simulink model "LKA"  (Simulink 7.9)
settings: Solver=ode23  StartTime=0.0  StopTime=tend  FixedStep=0.01  RelTol=1e-3
undefined symbols (not defined in the file or in its folder): pin
libraries: library x6, simulink x3
settings Model: Creator=Georg  LastModifiedBy=georgnestlinger
settings OptimizationCC: InlineParams=on
settings DebuggingCC: SolverPrmCheckMsg=none  FcnCallInpInsideContextMsg=Use local settings
settings GRTTargetCC: CombineOutputUpdateFcns=off  GRTInterface=on

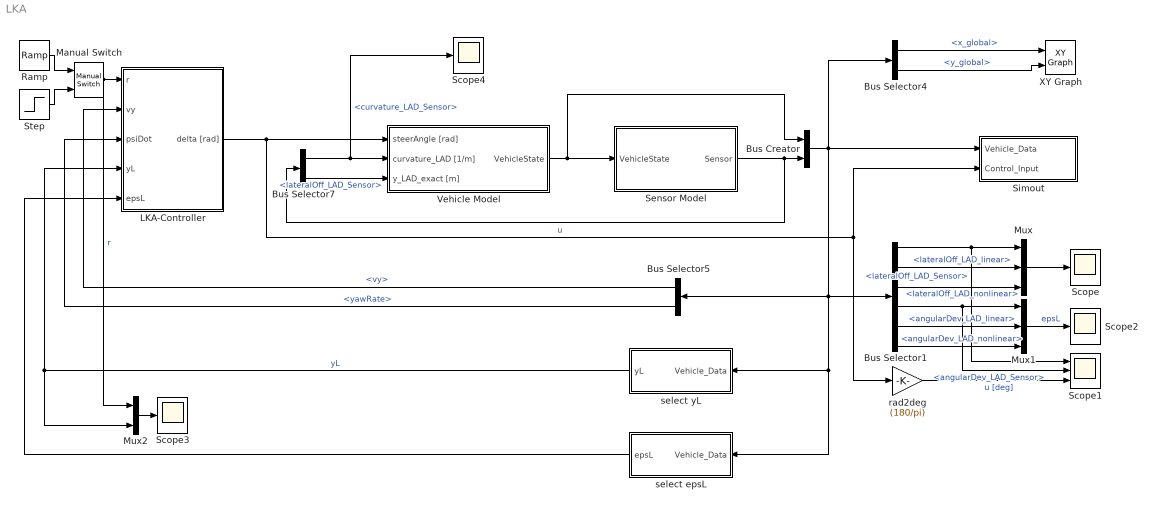
== system LKA ==
  Bus Creator : BusCreator  Inputs=2
  Bus Selector1 : BusSelector  OutputSignals=Sensor.lateralOff_LAD_Sensor,VehicleState.lateralOff_LAD_linear,VehicleState.lateralOff_LAD_nonlinear,Sensor.angularDev_LAD_Sensor,VehicleState.angularDev_LAD_linear,VehicleState.angularDev_LAD_nonlinear
  Bus Selector4 : BusSelector  OutputSignals=VehicleState.x_global,VehicleState.y_global
  Bus Selector5 : BusSelector  OutputSignals=VehicleState.vy,VehicleState.yawRate
  Bus Selector7 : BusSelector  OutputSignals=curvature_LAD_Sensor,lateralOff_LAD_Sensor
  LKA-Controller : Subsystem  BlockChoice=LQR
      settings: AttributesFormatString=%<BlockChoice>  TemplateBlock=library/LKA-Controller/LKA-Controller  MemberBlocks=AlgSynth,FKL,LQR,LQR_2int,ZR,ZR_2int
  Manual Switch : simulink/Signal Routing/Manual Switch  sw=0  action=0  varsize=off
  Mux : Mux  Inputs=3
  Mux1 : Mux  Inputs=3
  Mux2 : Mux  Inputs=2
  Ramp : simulink/Sources/Ramp  slope=1  start=8  X0=0
  Scope{,2..4} (4 alike) : Scope
      Scope settings: ShowLegends=on  YMin=-0.25  YMax=0.025  SaveName=ScopeData3
      Scope2 settings: TimeRange=13.0347  YMin=0.00932  YMax=0.009395
      Scope3 settings: TimeRange=5.66  YMin=0.999982  YMax=1  SaveName=ScopeData2
      Scope4 settings: TimeRange=13.0347  YMin=0.0019  YMax=0.0021  SaveName=ScopeData4
  Scope1 : Scope  NumInputPorts=3
      settings: TimeRange=13.0347  YMin=0~0~0  YMax=0.01~0.05~1
  Sensor Model : Subsystem
  Simout : Subsystem
  Step : Step  Time=10  SampleTime=0
  Vehicle Model : Subsystem
  XY Graph : simulink/Sinks/XY Graph  xmin=-50  xmax=700  ymin=-10  ymax=600  st=-1
  "rad2deg " : Gain  Gain=(180/pi)
  select epsL : Subsystem  BlockChoice=epsL_exactMdl
      settings: AttributesFormatString=%<BlockChoice>  TemplateBlock=library/LKA-Sensorik/select epsL  MemberBlocks=epsL_Sensor,epsL_exactMdl,epsL_linMdl
  select yL : Subsystem  BlockChoice=yL_Sensor
      settings: AttributesFormatString=%<BlockChoice>  TemplateBlock=library/LKA-Sensorik/select yL  MemberBlocks=yL_Sensor,yL_exactMdl,yL_linMdl
  wires:
  Bus Selector4/1 -> XY Graph/1  "<x_global>"
  Bus Selector4/2 -> XY Graph/2  "<y_global>"
  LKA-Controller/1(delta [rad]) -> Simout/2(Control_Input), "rad2deg "/1, Vehicle Model/1(steerAngle [rad])  "u"
  "rad2deg "/1 -> Scope1/3  "u [deg]"
  Bus Creator/1 -> Simout/1(Vehicle_Data), Bus Selector1/1, select epsL/1(Vehicle_Data), select yL/1(Vehicle_Data), Bus Selector5/1, Bus Selector4/1
  Step/1 -> Manual Switch/2
  Mux1/1 -> Scope2/1  "epsL"
  Manual Switch/1 -> LKA-Controller/1(r), Mux2/1  "r"
  Mux/1 -> Scope/1
  Bus Selector5/2 -> LKA-Controller/3(psiDot)  "<yawRate>"
  select yL/1(yL) -> Mux2/2, LKA-Controller/4(yL)  "yL"
  Bus Selector5/1 -> LKA-Controller/2(vy)  "<vy>"
  Bus Selector1/1 -> Mux/1, Scope1/1  "<lateralOff_LAD_Sensor>"
  Bus Selector1/2 -> Mux/2  "<lateralOff_LAD_linear>"
  Bus Selector1/3 -> Mux/3  "<lateralOff_LAD_nonlinear>"
  Bus Selector1/4 -> Mux1/1, Scope1/2  "<angularDev_LAD_Sensor>"
  Bus Selector1/5 -> Mux1/2  "<angularDev_LAD_linear>"
  Bus Selector1/6 -> Mux1/3  "<angularDev_LAD_nonlinear>"
  Sensor Model/1(Sensor) -> Bus Creator/2, Bus Selector7/1
  Vehicle Model/1(VehicleState) -> Bus Creator/1, Sensor Model/1(VehicleState)
  Bus Selector7/2 -> Vehicle Model/3(y_LAD_exact [m])  "<lateralOff_LAD_Sensor>"
  Bus Selector7/1 -> Scope4/1, Vehicle Model/2(curvature_LAD [1/m])  "<curvature_LAD_Sensor>"
  select epsL/1(epsL) -> LKA-Controller/5(epsL)
  Mux2/1 -> Scope3/1
  Ramp/1 -> Manual Switch/1

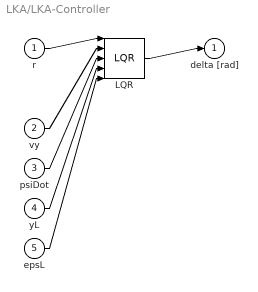
== system LKA/LKA-Controller ==
  r : Inport
  vy : Inport  Port=2
  psiDot : Inport  Port=3
  yL : Inport  Port=4
  epsL : Inport  Port=5
  LQR : library/LKA-Controller/LQR
  delta [rad] : Outport
  wires:
  r/1 -> LQR/1
  vy/1 -> LQR/2
  psiDot/1 -> LQR/3
  yL/1 -> LQR/4
  epsL/1 -> LQR/5
  LQR/1 -> delta [rad]/1

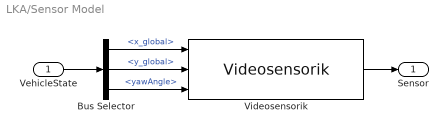
== system LKA/Sensor Model ==
  VehicleState : Inport
  Bus Selector : BusSelector  OutputSignals=x_global,y_global,yawAngle
  Videosensorik : library/LKA-Sensorik/Videosensorik
  Sensor : Outport
  wires:
  Videosensorik/1 -> Sensor/1
  VehicleState/1 -> Bus Selector/1
  Bus Selector/1 -> Videosensorik/1  "<x_global>"
  Bus Selector/2 -> Videosensorik/2  "<y_global>"
  Bus Selector/3 -> Videosensorik/3  "<yawAngle>"

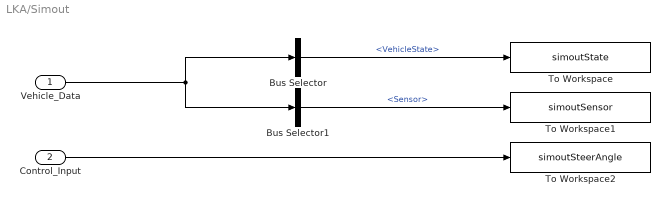
== system LKA/Simout ==
  Vehicle_Data : Inport
  Control_Input : Inport  Port=2
  Bus Selector : BusSelector  OutputSignals=VehicleState
  Bus Selector1 : BusSelector  OutputSignals=Sensor
  To Workspace : ToWorkspace  VariableName=simoutState  SampleTime=-1  SaveFormat=Structure With Time
  To Workspace1 : ToWorkspace  VariableName=simoutSensor  SampleTime=-1  SaveFormat=Structure With Time
  To Workspace2 : ToWorkspace  VariableName=simoutSteerAngle  SampleTime=-1  SaveFormat=Structure With Time
  wires:
  Vehicle_Data/1 -> Bus Selector1/1, Bus Selector/1
  Control_Input/1 -> To Workspace2/1
  Bus Selector/1 -> To Workspace/1  "<VehicleState>"
  Bus Selector1/1 -> To Workspace1/1  "<Sensor>"

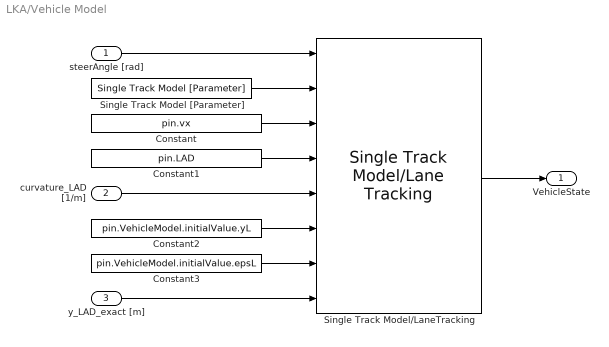
== system LKA/Vehicle Model ==
  steerAngle [rad] : Inport
  curvature_LAD [1/m] : Inport  Port=2
  y_LAD_exact [m] : Inport  Port=3
  Constant : Constant  Value=pin.vx
  Constant1 : Constant  Value=pin.LAD
  Constant2 : Constant  Value=pin.VehicleModel.initialValue.yL
  Constant3 : Constant  Value=pin.VehicleModel.initialValue.epsL
  Single Track Model [Parameter] : library/Vehicle Models/Single Track Models/Single Track Model [Parameter]  cs_front=pin.VehicleModel.parameter.csv  cs_rear=pin.VehicleModel.parameter.csh  l_front=pin.VehicleModel.parameter.lv  l_rear=pin.VehicleModel.parameter.lh  m=pin.VehicleModel.parameter.m  Izz=pin.VehicleModel.parameter.Iz
  Single Track Model/LaneTracking : library/Vehicle Models/Single Track Model//Lane Tracking
  VehicleState : Outport
  wires:
  Constant/1 -> Single Track Model/LaneTracking/3
  Constant1/1 -> Single Track Model/LaneTracking/4
  Constant2/1 -> Single Track Model/LaneTracking/6
  Constant3/1 -> Single Track Model/LaneTracking/7
  Single Track Model [Parameter]/1 -> Single Track Model/LaneTracking/2
  steerAngle [rad]/1 -> Single Track Model/LaneTracking/1
  curvature_LAD [1/m]/1 -> Single Track Model/LaneTracking/5
  y_LAD_exact [m]/1 -> Single Track Model/LaneTracking/8
  Single Track Model/LaneTracking/1 -> VehicleState/1

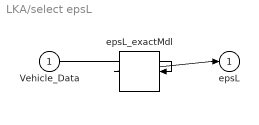
== system LKA/select epsL ==
  Vehicle_Data : Inport
  epsL_exactMdl : library/LKA-Sensorik/epsL_exactMdl
  epsL : Outport
  wires:
  Vehicle_Data/1 -> epsL_exactMdl/1
  epsL_exactMdl/1 -> epsL/1

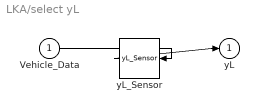
== system LKA/select yL ==
  Vehicle_Data : Inport
  yL_Sensor : library/LKA-Sensorik/yL_Sensor
  yL : Outport
  wires:
  Vehicle_Data/1 -> yL_Sensor/1
  yL_Sensor/1 -> yL/1
